simulink model "Lab2_PartA2"  (R2025b)
settings: Solver=VariableStepAuto  StartTime=0.0  StopTime=10.0  RelTol=1e-3
libraries: SignalEditorBlockLib x1
settings Model: Creator=Murl0  LastModifiedBy=Murl0

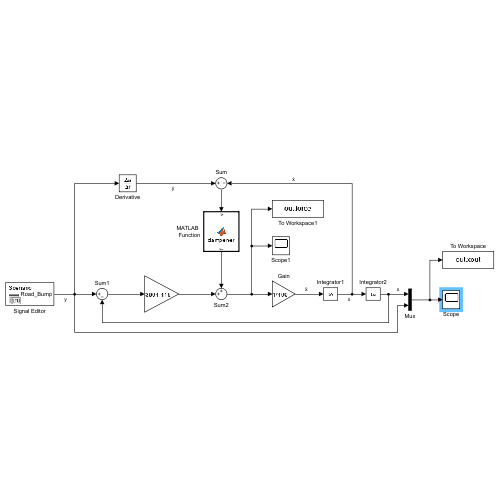
[thumbnail: Simulink's stored preview of the top-level diagram]
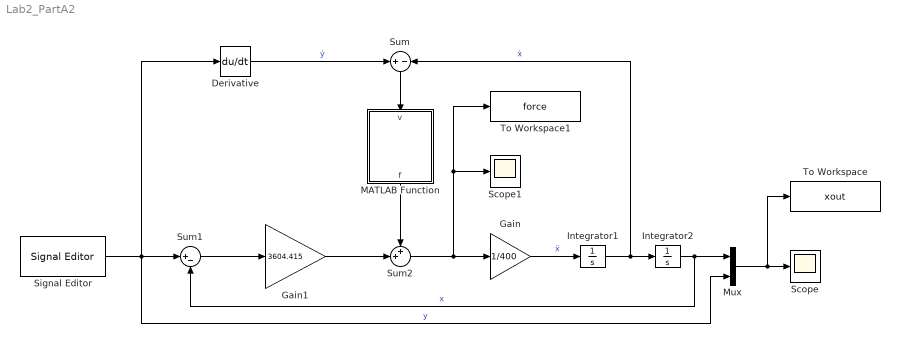
== system Lab2_PartA2 ==
  Derivative : Derivative
  Gain : Gain  Gain=1/400
  Gain1 : Gain  Gain=3604.415
  Integrator1 : Integrator
  Integrator2 : Integrator
  MATLAB Function : MATLAB Function  TreatAsAtomicUnit=on
  Mux : Mux  Inputs=2
  Scope : Scope
      settings: ActiveDisplayYMinimum=-1905.3217956620433  ActiveDisplayYMaximum=3789.9374150996618
  Scope1 : Scope
      settings: ActiveDisplayYMinimum=-1515.3241450529131  ActiveDisplayYMaximum=1384.2653234717261
  Signal Editor : SignalEditorBlockLib/Signal Editor  FileName=Input.mat  ActiveScenario=Scenario  ActiveSignal=Road_Bump  IsBus=off  OutputBusObjectStr=Bus: BusObject  SampleTime=0  ZeroCross=off  OutputAfterFinalValue=Setting to zero  Unit=m  PreserveSignalName=on  ApplySigPropsToAllScenarios=on  ApplySigPropsToAllSignals=off  SignalPropertySource=Dialog parameters
  Sum : Sum  Inputs=+-
  Sum1 : Sum  Inputs=|+-
  Sum2 : Sum  Inputs=++|
  To Workspace : ToWorkspace  VariableName=xout  SampleTime=-1
  To Workspace1 : ToWorkspace  VariableName=force  SampleTime=-1
  wires:
  Integrator2/1 -> Mux/1, Sum1/2  "x"
  Integrator1/1 -> Sum/2, Integrator2/1  "ẋ"
  Gain/1 -> Integrator1/1  "ẍ"
  MATLAB Function/1(f) -> Sum2/1
  Sum/1 -> MATLAB Function/1(v)
  Derivative/1 -> Sum/1  "ẏ"
  Gain1/1 -> Sum2/2
  Signal Editor/1 -> Derivative/1, Sum1/1, Mux/2  "y"
  Sum1/1 -> Gain1/1
  Mux/1 -> To Workspace/1, Scope/1
  Sum2/1 -> To Workspace1/1, Scope1/1, Gain/1

== matlab function Lab2_PartA2/MATLAB Function ==
  data: f output; v input
function f = dampener(v)
% Linear damper model
% Input: v = (ydot - xdot)
% Output: f = b * (ydot - xdot)

b = 84.056;   % Damping coefficient (N·s/m)
f = b * v;    % Linear damping force
end
